simulink model "myelectroMagnetModelStateSpace"  (R2020a)
settings: Solver=VariableStepAuto  StartTime=0.0  StopTime=5  RelTol=1e-3
undefined symbols (not defined in the file): Ax, Bx, Cx, Dx
settings Model: Creator=tanzc  LastModifiedBy=tanzc
settings DataIOCC: ReturnWorkspaceOutputs=off

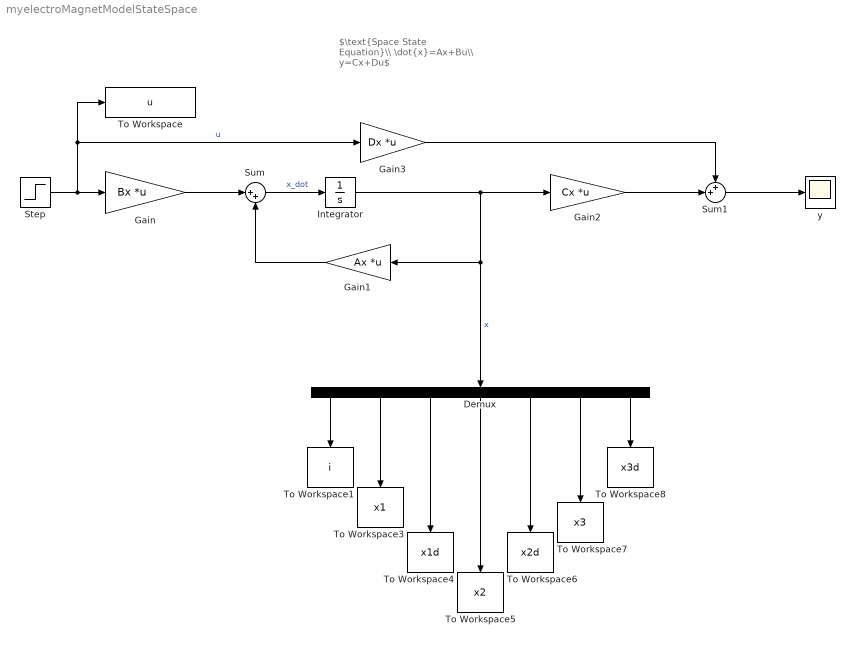
== system myelectroMagnetModelStateSpace ==
  note: $\text{Space State Equation}\\ \dot{x}=Ax+Bu\\ y=Cx+Du$
  Demux : Demux  Outputs=7
  Gain : Gain  Gain=Bx  Multiplication=Matrix(K*u) (u vector)
  Gain1 : Gain  Gain=Ax  Multiplication=Matrix(K*u) (u vector)
  Gain2 : Gain  Gain=Cx  Multiplication=Matrix(K*u) (u vector)
  Gain3 : Gain  Gain=Dx  Multiplication=Matrix(K*u) (u vector)
  Integrator : Integrator
  Step : Step  SampleTime=0
  Sum : Sum  Inputs=|++
  Sum1 : Sum  Inputs=++|
  To Workspace : ToWorkspace  VariableName=u  SaveFormat=Timeseries  SampleTime=-1
  To Workspace1 : ToWorkspace  VariableName=i  SaveFormat=Timeseries  SampleTime=-1
  To Workspace3 : ToWorkspace  VariableName=x1  SaveFormat=Timeseries  SampleTime=-1
  To Workspace4 : ToWorkspace  VariableName=x1d  SaveFormat=Timeseries  SampleTime=-1
  To Workspace5 : ToWorkspace  VariableName=x2  SaveFormat=Timeseries  SampleTime=-1
  To Workspace6 : ToWorkspace  VariableName=x2d  SaveFormat=Timeseries  SampleTime=-1
  To Workspace7 : ToWorkspace  VariableName=x3  SaveFormat=Timeseries  SampleTime=-1
  To Workspace8 : ToWorkspace  VariableName=x3d  SaveFormat=Timeseries  SampleTime=-1
  y : Scope
  wires:
  Integrator/1 -> Demux/1, Gain1/1, Gain2/1  "x"
  Step/1 -> To Workspace/1, Gain3/1, Gain/1  "u"
  Sum/1 -> Integrator/1  "x_dot"
  Gain/1 -> Sum/1
  Gain1/1 -> Sum/2
  Gain2/1 -> Sum1/2
  Gain3/1 -> Sum1/1
  Sum1/1 -> y/1
  Demux/1 -> To Workspace1/1
  Demux/3 -> To Workspace4/1
  Demux/2 -> To Workspace3/1
  Demux/4 -> To Workspace5/1
  Demux/5 -> To Workspace6/1
  Demux/6 -> To Workspace7/1
  Demux/7 -> To Workspace8/1
